simulink model "gm_FP_sub"  (R2023a)
settings: Solver=FixedStepAuto  StartTime=0.0  StopTime=T  RelTol=1e-3  EnableMultiTasking=on
undefined symbols (not defined in the file or in its folder): Ts
libraries: My_FI_Operations x114, simulink x1
(part 2 of 2)

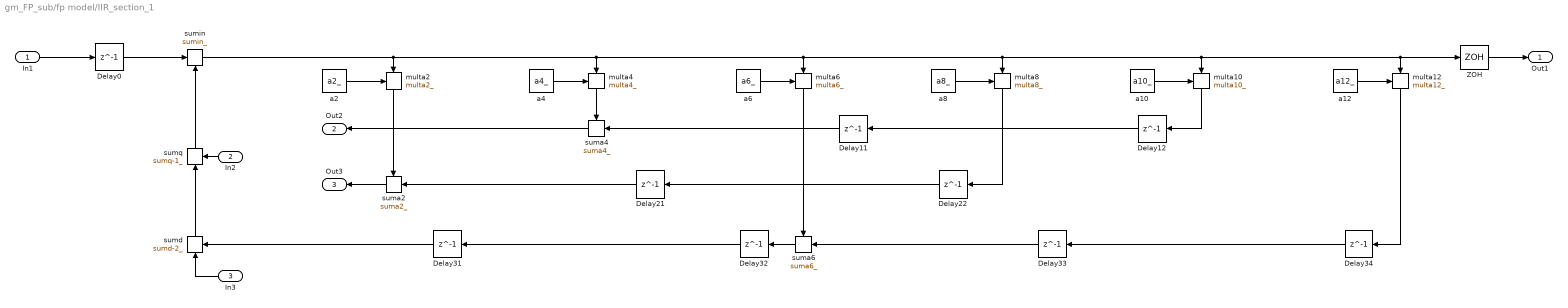
== system gm_FP_sub/fp model/IIR_section_1 ==
  In1 : Inport
  In2 : Inport  Port=2
  In3 : Inport  Port=3
  Delay{0,11..12,21..22,31..34} (9 alike) : Delay  DelayLength=1  SampleTime=3*Ts
  ZOH : ZeroOrderHold  SampleTime=3*Ts
  a10 : My_FI_Operations/a10_  SystemSampleTime=-1  VariantActivationTime=update diagram  Latency=0  AutoFrameSizeCalculation=off
  a12 : My_FI_Operations/a12_  SystemSampleTime=-1  VariantActivationTime=update diagram  Latency=0  AutoFrameSizeCalculation=off
  a2 : My_FI_Operations/a2_  SystemSampleTime=-1  VariantActivationTime=update diagram  Latency=0  AutoFrameSizeCalculation=off
  a4 : My_FI_Operations/a4_  SystemSampleTime=-1  VariantActivationTime=update diagram  Latency=0  AutoFrameSizeCalculation=off
  a6 : My_FI_Operations/a6_  SystemSampleTime=-1  VariantActivationTime=update diagram  Latency=0  AutoFrameSizeCalculation=off
  a8 : My_FI_Operations/a8_  SystemSampleTime=-1  VariantActivationTime=update diagram  Latency=0  AutoFrameSizeCalculation=off
  multa10 : My_FI_Operations/multa10_  SystemSampleTime=-1  VariantActivationTime=update diagram  Latency=0  AutoFrameSizeCalculation=off
      settings: PortSchema="{\"entries\":[{\"content\":{\"sides\":[{\"content\":{\"connectorIds\":[\"In1\"]},\"type\":\"ConnectorPlacement.EquallySpacedRectSide\",\"uuid\":\"423828e0-6700-4575-ac06-a5fb7cb5569f\"},{\"content\":{\"connectorIds\":[],\"side\":\"RIGHT\"},\"type\":\"ConnectorPlacement.EquallySpacedRectSide\",\"uuid\":\"a42db842-eb55-44f2-8f04-0144bc45d908\"},{\"content\":{\"connectorIds\":[\"In2\"],\"side\":\"TOP\"},\"type\":\"ConnectorPlacement.EquallySpacedRectSide\",\"uuid\":\"eef5137d-31f0-46b4-a53b-5aa31464a7f9\"},{\"content\":{\"connectorIds\":[\"Out1\"],\"side\":\"BOTTOM\"},\"type\":\"ConnectorPlacement.EquallySpacedRectSide\",\"uuid\":\"0c804fa9-8d94-49f3-91d8-5fb511150c33\"}]},\"type\":\"ConnectorPlacement.EquallySpacedConnector\",\"uuid\":\"7dd7fe03-b221-4701-a7b2-6552f08320da\"}],\"packageUris\":[\"http://schema.mathworks.com/mf0/Connector/R2020b\"],\"version\":\"1.0\"}"
  multa12 : My_FI_Operations/multa12_  SystemSampleTime=-1  VariantActivationTime=update diagram  Latency=0  AutoFrameSizeCalculation=off
      settings: PortSchema="{\"entries\":[{\"content\":{\"sides\":[{\"content\":{\"connectorIds\":[\"In1\"]},\"type\":\"ConnectorPlacement.EquallySpacedRectSide\",\"uuid\":\"423828e0-6700-4575-ac06-a5fb7cb5569f\"},{\"content\":{\"connectorIds\":[],\"side\":\"RIGHT\"},\"type\":\"ConnectorPlacement.EquallySpacedRectSide\",\"uuid\":\"a42db842-eb55-44f2-8f04-0144bc45d908\"},{\"content\":{\"connectorIds\":[\"In2\"],\"side\":\"TOP\"},\"type\":\"ConnectorPlacement.EquallySpacedRectSide\",\"uuid\":\"eef5137d-31f0-46b4-a53b-5aa31464a7f9\"},{\"content\":{\"connectorIds\":[\"Out1\"],\"side\":\"BOTTOM\"},\"type\":\"ConnectorPlacement.EquallySpacedRectSide\",\"uuid\":\"8449918d-02c6-4967-8b4f-9e277713318d\"}]},\"type\":\"ConnectorPlacement.EquallySpacedConnector\",\"uuid\":\"7dd7fe03-b221-4701-a7b2-6552f08320da\"}],\"packageUris\":[\"http://schema.mathworks.com/mf0/Connector/R2020b\"],\"version\":\"1.0\"}"
  multa2 : My_FI_Operations/multa2_  SystemSampleTime=-1  VariantActivationTime=update diagram  Latency=0  AutoFrameSizeCalculation=off
      settings: PortSchema="{\"entries\":[{\"content\":{\"sides\":[{\"content\":{\"connectorIds\":[\"In1\"]},\"type\":\"ConnectorPlacement.EquallySpacedRectSide\",\"uuid\":\"423828e0-6700-4575-ac06-a5fb7cb5569f\"},{\"content\":{\"connectorIds\":[],\"side\":\"RIGHT\"},\"type\":\"ConnectorPlacement.EquallySpacedRectSide\",\"uuid\":\"a42db842-eb55-44f2-8f04-0144bc45d908\"},{\"content\":{\"connectorIds\":[\"In2\"],\"side\":\"TOP\"},\"type\":\"ConnectorPlacement.EquallySpacedRectSide\",\"uuid\":\"eef5137d-31f0-46b4-a53b-5aa31464a7f9\"},{\"content\":{\"connectorIds\":[\"Out1\"],\"side\":\"BOTTOM\"},\"type\":\"ConnectorPlacement.EquallySpacedRectSide\",\"uuid\":\"55d96b2a-2b7e-4fdf-a401-8e78f7d2a1aa\"}]},\"type\":\"ConnectorPlacement.EquallySpacedConnector\",\"uuid\":\"7dd7fe03-b221-4701-a7b2-6552f08320da\"}],\"packageUris\":[\"http://schema.mathworks.com/mf0/Connector/R2020b\"],\"version\":\"1.0\"}"
  multa4 : My_FI_Operations/multa4_  SystemSampleTime=-1  VariantActivationTime=update diagram  Latency=0  AutoFrameSizeCalculation=off
      settings: PortSchema="{\"entries\":[{\"content\":{\"sides\":[{\"content\":{\"connectorIds\":[\"In1\"]},\"type\":\"ConnectorPlacement.EquallySpacedRectSide\",\"uuid\":\"423828e0-6700-4575-ac06-a5fb7cb5569f\"},{\"content\":{\"connectorIds\":[],\"side\":\"RIGHT\"},\"type\":\"ConnectorPlacement.EquallySpacedRectSide\",\"uuid\":\"a42db842-eb55-44f2-8f04-0144bc45d908\"},{\"content\":{\"connectorIds\":[\"In2\"],\"side\":\"TOP\"},\"type\":\"ConnectorPlacement.EquallySpacedRectSide\",\"uuid\":\"eef5137d-31f0-46b4-a53b-5aa31464a7f9\"},{\"content\":{\"connectorIds\":[\"Out1\"],\"side\":\"BOTTOM\"},\"type\":\"ConnectorPlacement.EquallySpacedRectSide\",\"uuid\":\"24a9476e-4370-431a-bbc5-245c90c7a6e7\"}]},\"type\":\"ConnectorPlacement.EquallySpacedConnector\",\"uuid\":\"7dd7fe03-b221-4701-a7b2-6552f08320da\"}],\"packageUris\":[\"http://schema.mathworks.com/mf0/Connector/R2020b\"],\"version\":\"1.0\"}"
  multa6 : My_FI_Operations/multa6_  SystemSampleTime=-1  VariantActivationTime=update diagram  Latency=0  AutoFrameSizeCalculation=off
      settings: PortSchema="{\"entries\":[{\"content\":{\"sides\":[{\"content\":{\"connectorIds\":[\"In1\"]},\"type\":\"ConnectorPlacement.EquallySpacedRectSide\",\"uuid\":\"423828e0-6700-4575-ac06-a5fb7cb5569f\"},{\"content\":{\"connectorIds\":[],\"side\":\"RIGHT\"},\"type\":\"ConnectorPlacement.EquallySpacedRectSide\",\"uuid\":\"a42db842-eb55-44f2-8f04-0144bc45d908\"},{\"content\":{\"connectorIds\":[\"In2\"],\"side\":\"TOP\"},\"type\":\"ConnectorPlacement.EquallySpacedRectSide\",\"uuid\":\"eef5137d-31f0-46b4-a53b-5aa31464a7f9\"},{\"content\":{\"connectorIds\":[\"Out1\"],\"side\":\"BOTTOM\"},\"type\":\"ConnectorPlacement.EquallySpacedRectSide\",\"uuid\":\"47329aef-84bb-47a0-9b32-b12909a392a1\"}]},\"type\":\"ConnectorPlacement.EquallySpacedConnector\",\"uuid\":\"7dd7fe03-b221-4701-a7b2-6552f08320da\"}],\"packageUris\":[\"http://schema.mathworks.com/mf0/Connector/R2020b\"],\"version\":\"1.0\"}"
  multa8 : My_FI_Operations/multa8_  SystemSampleTime=-1  VariantActivationTime=update diagram  Latency=0  AutoFrameSizeCalculation=off
      settings: PortSchema="{\"entries\":[{\"content\":{\"sides\":[{\"content\":{\"connectorIds\":[\"In1\"]},\"type\":\"ConnectorPlacement.EquallySpacedRectSide\",\"uuid\":\"423828e0-6700-4575-ac06-a5fb7cb5569f\"},{\"content\":{\"connectorIds\":[],\"side\":\"RIGHT\"},\"type\":\"ConnectorPlacement.EquallySpacedRectSide\",\"uuid\":\"a42db842-eb55-44f2-8f04-0144bc45d908\"},{\"content\":{\"connectorIds\":[\"In2\"],\"side\":\"TOP\"},\"type\":\"ConnectorPlacement.EquallySpacedRectSide\",\"uuid\":\"eef5137d-31f0-46b4-a53b-5aa31464a7f9\"},{\"content\":{\"connectorIds\":[\"Out1\"],\"side\":\"BOTTOM\"},\"type\":\"ConnectorPlacement.EquallySpacedRectSide\",\"uuid\":\"5c073f60-f22f-4cd7-abc5-d0d5f88f0213\"}]},\"type\":\"ConnectorPlacement.EquallySpacedConnector\",\"uuid\":\"7dd7fe03-b221-4701-a7b2-6552f08320da\"}],\"packageUris\":[\"http://schema.mathworks.com/mf0/Connector/R2020b\"],\"version\":\"1.0\"}"
  suma2 : My_FI_Operations/suma2_  SystemSampleTime=-1  VariantActivationTime=update diagram  Latency=0  AutoFrameSizeCalculation=off
      settings: PortSchema="{\"entries\":[{\"content\":{\"sides\":[{\"content\":{\"connectorIds\":[\"Out1\"]},\"type\":\"ConnectorPlacement.EquallySpacedRectSide\",\"uuid\":\"423828e0-6700-4575-ac06-a5fb7cb5569f\"},{\"content\":{\"connectorIds\":[\"In2\"],\"side\":\"RIGHT\"},\"type\":\"ConnectorPlacement.EquallySpacedRectSide\",\"uuid\":\"a42db842-eb55-44f2-8f04-0144bc45d908\"},{\"content\":{\"connectorIds\":[\"In1\"],\"side\":\"TOP\"},\"type\":\"ConnectorPlacement.EquallySpacedRectSide\",\"uuid\":\"eef5137d-31f0-46b4-a53b-5aa31464a7f9\"}]},\"type\":\"ConnectorPlacement.EquallySpacedConnector\",\"uuid\":\"7dd7fe03-b221-4701-a7b2-6552f08320da\"}],\"packageUris\":[\"http://schema.mathworks.com/mf0/Connector/R2020b\"],\"version\":\"1.0\"}"
  suma4 : My_FI_Operations/suma4_  SystemSampleTime=-1  VariantActivationTime=update diagram  Latency=0  AutoFrameSizeCalculation=off
      settings: PortSchema="{\"entries\":[{\"content\":{\"sides\":[{\"content\":{\"connectorIds\":[\"Out1\"]},\"type\":\"ConnectorPlacement.EquallySpacedRectSide\",\"uuid\":\"423828e0-6700-4575-ac06-a5fb7cb5569f\"},{\"content\":{\"connectorIds\":[\"In2\"],\"side\":\"RIGHT\"},\"type\":\"ConnectorPlacement.EquallySpacedRectSide\",\"uuid\":\"a42db842-eb55-44f2-8f04-0144bc45d908\"},{\"content\":{\"connectorIds\":[\"In1\"],\"side\":\"TOP\"},\"type\":\"ConnectorPlacement.EquallySpacedRectSide\",\"uuid\":\"eef5137d-31f0-46b4-a53b-5aa31464a7f9\"}]},\"type\":\"ConnectorPlacement.EquallySpacedConnector\",\"uuid\":\"7dd7fe03-b221-4701-a7b2-6552f08320da\"}],\"packageUris\":[\"http://schema.mathworks.com/mf0/Connector/R2020b\"],\"version\":\"1.0\"}"
  suma6 : My_FI_Operations/suma6_  SystemSampleTime=-1  VariantActivationTime=update diagram  Latency=0  AutoFrameSizeCalculation=off
      settings: PortSchema="{\"entries\":[{\"content\":{\"sides\":[{\"content\":{\"connectorIds\":[\"Out1\"]},\"type\":\"ConnectorPlacement.EquallySpacedRectSide\",\"uuid\":\"423828e0-6700-4575-ac06-a5fb7cb5569f\"},{\"content\":{\"connectorIds\":[\"In2\"],\"side\":\"RIGHT\"},\"type\":\"ConnectorPlacement.EquallySpacedRectSide\",\"uuid\":\"a42db842-eb55-44f2-8f04-0144bc45d908\"},{\"content\":{\"connectorIds\":[\"In1\"],\"side\":\"TOP\"},\"type\":\"ConnectorPlacement.EquallySpacedRectSide\",\"uuid\":\"eef5137d-31f0-46b4-a53b-5aa31464a7f9\"}]},\"type\":\"ConnectorPlacement.EquallySpacedConnector\",\"uuid\":\"7dd7fe03-b221-4701-a7b2-6552f08320da\"}],\"packageUris\":[\"http://schema.mathworks.com/mf0/Connector/R2020b\"],\"version\":\"1.0\"}"
  sumd : My_FI_Operations/sumd-2_  SystemSampleTime=-1  VariantActivationTime=update diagram  Latency=0  AutoFrameSizeCalculation=off
      settings: PortSchema="{\"entries\":[{\"content\":{\"sides\":[{\"content\":{\"connectorIds\":[]},\"type\":\"ConnectorPlacement.EquallySpacedRectSide\",\"uuid\":\"423828e0-6700-4575-ac06-a5fb7cb5569f\"},{\"content\":{\"connectorIds\":[\"In2\"],\"side\":\"RIGHT\"},\"type\":\"ConnectorPlacement.EquallySpacedRectSide\",\"uuid\":\"a42db842-eb55-44f2-8f04-0144bc45d908\"},{\"content\":{\"connectorIds\":[\"Out1\"],\"side\":\"TOP\"},\"type\":\"ConnectorPlacement.EquallySpacedRectSide\",\"uuid\":\"eef5137d-31f0-46b4-a53b-5aa31464a7f9\"},{\"content\":{\"connectorIds\":[\"In1\"],\"side\":\"BOTTOM\"},\"type\":\"ConnectorPlacement.EquallySpacedRectSide\",\"uuid\":\"0a29e77a-4bdf-45d0-8a25-1103c3446174\"}]},\"type\":\"ConnectorPlacement.EquallySpacedConnector\",\"uuid\":\"7dd7fe03-b221-4701-a7b2-6552f08320da\"}],\"packageUris\":[\"http://schema.mathworks.com/mf0/Connector/R2020b\"],\"version\":\"1.0\"}"
  sumin : My_FI_Operations/sumin_  SystemSampleTime=-1  VariantActivationTime=update diagram  Latency=0  AutoFrameSizeCalculation=off
      settings: PortSchema="{\"entries\":[{\"content\":{\"sides\":[{\"content\":{\"connectorIds\":[\"In1\"]},\"type\":\"ConnectorPlacement.EquallySpacedRectSide\",\"uuid\":\"423828e0-6700-4575-ac06-a5fb7cb5569f\"},{\"content\":{\"connectorIds\":[\"Out1\"],\"side\":\"RIGHT\"},\"type\":\"ConnectorPlacement.EquallySpacedRectSide\",\"uuid\":\"a42db842-eb55-44f2-8f04-0144bc45d908\"},{\"content\":{\"connectorIds\":[],\"side\":\"TOP\"},\"type\":\"ConnectorPlacement.EquallySpacedRectSide\",\"uuid\":\"eef5137d-31f0-46b4-a53b-5aa31464a7f9\"},{\"content\":{\"connectorIds\":[\"In2\"],\"side\":\"BOTTOM\"},\"type\":\"ConnectorPlacement.EquallySpacedRectSide\",\"uuid\":\"f3760898-0e2b-4385-8757-2cc61988fa54\"}]},\"type\":\"ConnectorPlacement.EquallySpacedConnector\",\"uuid\":\"7dd7fe03-b221-4701-a7b2-6552f08320da\"}],\"packageUris\":[\"http://schema.mathworks.com/mf0/Connector/R2020b\"],\"version\":\"1.0\"}"
  sumq : My_FI_Operations/sumq-1_  SystemSampleTime=-1  VariantActivationTime=update diagram  Latency=0  AutoFrameSizeCalculation=off
      settings: PortSchema="{\"entries\":[{\"content\":{\"sides\":[{\"content\":{\"connectorIds\":[]},\"type\":\"ConnectorPlacement.EquallySpacedRectSide\",\"uuid\":\"423828e0-6700-4575-ac06-a5fb7cb5569f\"},{\"content\":{\"connectorIds\":[\"In2\"],\"side\":\"RIGHT\"},\"type\":\"ConnectorPlacement.EquallySpacedRectSide\",\"uuid\":\"a42db842-eb55-44f2-8f04-0144bc45d908\"},{\"content\":{\"connectorIds\":[\"Out1\"],\"side\":\"TOP\"},\"type\":\"ConnectorPlacement.EquallySpacedRectSide\",\"uuid\":\"eef5137d-31f0-46b4-a53b-5aa31464a7f9\"},{\"content\":{\"connectorIds\":[\"In1\"],\"side\":\"BOTTOM\"},\"type\":\"ConnectorPlacement.EquallySpacedRectSide\",\"uuid\":\"2873f229-5340-47da-9b40-109923f96826\"}]},\"type\":\"ConnectorPlacement.EquallySpacedConnector\",\"uuid\":\"7dd7fe03-b221-4701-a7b2-6552f08320da\"}],\"packageUris\":[\"http://schema.mathworks.com/mf0/Connector/R2020b\"],\"version\":\"1.0\"}"
  Out1 : Outport
  Out2 : Outport  Port=2
  Out3 : Outport  Port=3
  wires:
  suma4/1 -> Out2/1
  suma2/1 -> Out3/1
  In3/1 -> sumd/1
  In1/1 -> Delay0/1
  In2/1 -> sumq/2
  a6/1 -> multa6/1
  sumq/1 -> sumin/2
  multa8/1 -> Delay22/1
  multa10/1 -> Delay12/1
  Delay11/1 -> suma4/2
  suma6/1 -> Delay32/1
  a8/1 -> multa8/1
  Delay34/1 -> Delay33/1
  multa2/1 -> suma2/1
  multa12/1 -> Delay34/1
  a4/1 -> multa4/1
  a10/1 -> multa10/1
  multa6/1 -> suma6/1
  ZOH/1 -> Out1/1
  Delay12/1 -> Delay11/1
  multa4/1 -> suma4/1
  a2/1 -> multa2/1
  sumd/1 -> sumq/1
  Delay21/1 -> suma2/2
  Delay32/1 -> Delay31/1
  Delay33/1 -> suma6/2
  sumin/1 -> ZOH/1, multa12/2, multa10/2, multa8/2, multa6/2, multa4/2, multa2/2
  Delay31/1 -> sumd/2
  Delay22/1 -> Delay21/1
  a12/1 -> multa12/1
  Delay0/1 -> sumin/1

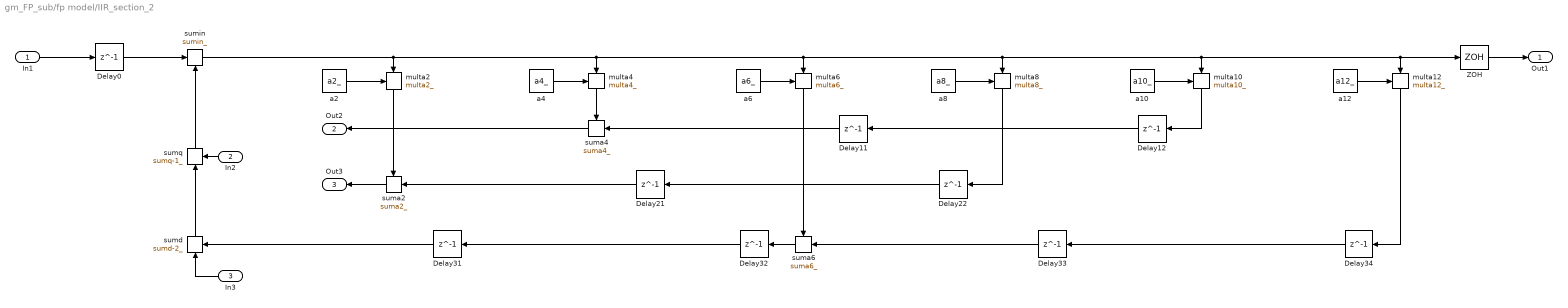
== system gm_FP_sub/fp model/IIR_section_2 ==
  In1 : Inport
  In2 : Inport  Port=2
  In3 : Inport  Port=3
  Delay{0,11..12,21..22,31..34} (9 alike) : Delay  DelayLength=1  SampleTime=3*Ts
  ZOH : ZeroOrderHold  SampleTime=3*Ts
  a10 : My_FI_Operations/a10_  SystemSampleTime=-1  VariantActivationTime=update diagram  Latency=0  AutoFrameSizeCalculation=off
  a12 : My_FI_Operations/a12_  SystemSampleTime=-1  VariantActivationTime=update diagram  Latency=0  AutoFrameSizeCalculation=off
  a2 : My_FI_Operations/a2_  SystemSampleTime=-1  VariantActivationTime=update diagram  Latency=0  AutoFrameSizeCalculation=off
  a4 : My_FI_Operations/a4_  SystemSampleTime=-1  VariantActivationTime=update diagram  Latency=0  AutoFrameSizeCalculation=off
  a6 : My_FI_Operations/a6_  SystemSampleTime=-1  VariantActivationTime=update diagram  Latency=0  AutoFrameSizeCalculation=off
  a8 : My_FI_Operations/a8_  SystemSampleTime=-1  VariantActivationTime=update diagram  Latency=0  AutoFrameSizeCalculation=off
  multa10 : My_FI_Operations/multa10_  SystemSampleTime=-1  VariantActivationTime=update diagram  Latency=0  AutoFrameSizeCalculation=off
      settings: PortSchema="{\"entries\":[{\"content\":{\"sides\":[{\"content\":{\"connectorIds\":[\"In1\"]},\"type\":\"ConnectorPlacement.EquallySpacedRectSide\",\"uuid\":\"423828e0-6700-4575-ac06-a5fb7cb5569f\"},{\"content\":{\"connectorIds\":[],\"side\":\"RIGHT\"},\"type\":\"ConnectorPlacement.EquallySpacedRectSide\",\"uuid\":\"a42db842-eb55-44f2-8f04-0144bc45d908\"},{\"content\":{\"connectorIds\":[\"In2\"],\"side\":\"TOP\"},\"type\":\"ConnectorPlacement.EquallySpacedRectSide\",\"uuid\":\"eef5137d-31f0-46b4-a53b-5aa31464a7f9\"},{\"content\":{\"connectorIds\":[\"Out1\"],\"side\":\"BOTTOM\"},\"type\":\"ConnectorPlacement.EquallySpacedRectSide\",\"uuid\":\"0c804fa9-8d94-49f3-91d8-5fb511150c33\"}]},\"type\":\"ConnectorPlacement.EquallySpacedConnector\",\"uuid\":\"7dd7fe03-b221-4701-a7b2-6552f08320da\"}],\"packageUris\":[\"http://schema.mathworks.com/mf0/Connector/R2020b\"],\"version\":\"1.0\"}"
  multa12 : My_FI_Operations/multa12_  SystemSampleTime=-1  VariantActivationTime=update diagram  Latency=0  AutoFrameSizeCalculation=off
      settings: PortSchema="{\"entries\":[{\"content\":{\"sides\":[{\"content\":{\"connectorIds\":[\"In1\"]},\"type\":\"ConnectorPlacement.EquallySpacedRectSide\",\"uuid\":\"423828e0-6700-4575-ac06-a5fb7cb5569f\"},{\"content\":{\"connectorIds\":[],\"side\":\"RIGHT\"},\"type\":\"ConnectorPlacement.EquallySpacedRectSide\",\"uuid\":\"a42db842-eb55-44f2-8f04-0144bc45d908\"},{\"content\":{\"connectorIds\":[\"In2\"],\"side\":\"TOP\"},\"type\":\"ConnectorPlacement.EquallySpacedRectSide\",\"uuid\":\"eef5137d-31f0-46b4-a53b-5aa31464a7f9\"},{\"content\":{\"connectorIds\":[\"Out1\"],\"side\":\"BOTTOM\"},\"type\":\"ConnectorPlacement.EquallySpacedRectSide\",\"uuid\":\"8449918d-02c6-4967-8b4f-9e277713318d\"}]},\"type\":\"ConnectorPlacement.EquallySpacedConnector\",\"uuid\":\"7dd7fe03-b221-4701-a7b2-6552f08320da\"}],\"packageUris\":[\"http://schema.mathworks.com/mf0/Connector/R2020b\"],\"version\":\"1.0\"}"
  multa2 : My_FI_Operations/multa2_  SystemSampleTime=-1  VariantActivationTime=update diagram  Latency=0  AutoFrameSizeCalculation=off
      settings: PortSchema="{\"entries\":[{\"content\":{\"sides\":[{\"content\":{\"connectorIds\":[\"In1\"]},\"type\":\"ConnectorPlacement.EquallySpacedRectSide\",\"uuid\":\"423828e0-6700-4575-ac06-a5fb7cb5569f\"},{\"content\":{\"connectorIds\":[],\"side\":\"RIGHT\"},\"type\":\"ConnectorPlacement.EquallySpacedRectSide\",\"uuid\":\"a42db842-eb55-44f2-8f04-0144bc45d908\"},{\"content\":{\"connectorIds\":[\"In2\"],\"side\":\"TOP\"},\"type\":\"ConnectorPlacement.EquallySpacedRectSide\",\"uuid\":\"eef5137d-31f0-46b4-a53b-5aa31464a7f9\"},{\"content\":{\"connectorIds\":[\"Out1\"],\"side\":\"BOTTOM\"},\"type\":\"ConnectorPlacement.EquallySpacedRectSide\",\"uuid\":\"55d96b2a-2b7e-4fdf-a401-8e78f7d2a1aa\"}]},\"type\":\"ConnectorPlacement.EquallySpacedConnector\",\"uuid\":\"7dd7fe03-b221-4701-a7b2-6552f08320da\"}],\"packageUris\":[\"http://schema.mathworks.com/mf0/Connector/R2020b\"],\"version\":\"1.0\"}"
  multa4 : My_FI_Operations/multa4_  SystemSampleTime=-1  VariantActivationTime=update diagram  Latency=0  AutoFrameSizeCalculation=off
      settings: PortSchema="{\"entries\":[{\"content\":{\"sides\":[{\"content\":{\"connectorIds\":[\"In1\"]},\"type\":\"ConnectorPlacement.EquallySpacedRectSide\",\"uuid\":\"423828e0-6700-4575-ac06-a5fb7cb5569f\"},{\"content\":{\"connectorIds\":[],\"side\":\"RIGHT\"},\"type\":\"ConnectorPlacement.EquallySpacedRectSide\",\"uuid\":\"a42db842-eb55-44f2-8f04-0144bc45d908\"},{\"content\":{\"connectorIds\":[\"In2\"],\"side\":\"TOP\"},\"type\":\"ConnectorPlacement.EquallySpacedRectSide\",\"uuid\":\"eef5137d-31f0-46b4-a53b-5aa31464a7f9\"},{\"content\":{\"connectorIds\":[\"Out1\"],\"side\":\"BOTTOM\"},\"type\":\"ConnectorPlacement.EquallySpacedRectSide\",\"uuid\":\"24a9476e-4370-431a-bbc5-245c90c7a6e7\"}]},\"type\":\"ConnectorPlacement.EquallySpacedConnector\",\"uuid\":\"7dd7fe03-b221-4701-a7b2-6552f08320da\"}],\"packageUris\":[\"http://schema.mathworks.com/mf0/Connector/R2020b\"],\"version\":\"1.0\"}"
  multa6 : My_FI_Operations/multa6_  SystemSampleTime=-1  VariantActivationTime=update diagram  Latency=0  AutoFrameSizeCalculation=off
      settings: PortSchema="{\"entries\":[{\"content\":{\"sides\":[{\"content\":{\"connectorIds\":[\"In1\"]},\"type\":\"ConnectorPlacement.EquallySpacedRectSide\",\"uuid\":\"423828e0-6700-4575-ac06-a5fb7cb5569f\"},{\"content\":{\"connectorIds\":[],\"side\":\"RIGHT\"},\"type\":\"ConnectorPlacement.EquallySpacedRectSide\",\"uuid\":\"a42db842-eb55-44f2-8f04-0144bc45d908\"},{\"content\":{\"connectorIds\":[\"In2\"],\"side\":\"TOP\"},\"type\":\"ConnectorPlacement.EquallySpacedRectSide\",\"uuid\":\"eef5137d-31f0-46b4-a53b-5aa31464a7f9\"},{\"content\":{\"connectorIds\":[\"Out1\"],\"side\":\"BOTTOM\"},\"type\":\"ConnectorPlacement.EquallySpacedRectSide\",\"uuid\":\"47329aef-84bb-47a0-9b32-b12909a392a1\"}]},\"type\":\"ConnectorPlacement.EquallySpacedConnector\",\"uuid\":\"7dd7fe03-b221-4701-a7b2-6552f08320da\"}],\"packageUris\":[\"http://schema.mathworks.com/mf0/Connector/R2020b\"],\"version\":\"1.0\"}"
  multa8 : My_FI_Operations/multa8_  SystemSampleTime=-1  VariantActivationTime=update diagram  Latency=0  AutoFrameSizeCalculation=off
      settings: PortSchema="{\"entries\":[{\"content\":{\"sides\":[{\"content\":{\"connectorIds\":[\"In1\"]},\"type\":\"ConnectorPlacement.EquallySpacedRectSide\",\"uuid\":\"423828e0-6700-4575-ac06-a5fb7cb5569f\"},{\"content\":{\"connectorIds\":[],\"side\":\"RIGHT\"},\"type\":\"ConnectorPlacement.EquallySpacedRectSide\",\"uuid\":\"a42db842-eb55-44f2-8f04-0144bc45d908\"},{\"content\":{\"connectorIds\":[\"In2\"],\"side\":\"TOP\"},\"type\":\"ConnectorPlacement.EquallySpacedRectSide\",\"uuid\":\"eef5137d-31f0-46b4-a53b-5aa31464a7f9\"},{\"content\":{\"connectorIds\":[\"Out1\"],\"side\":\"BOTTOM\"},\"type\":\"ConnectorPlacement.EquallySpacedRectSide\",\"uuid\":\"5c073f60-f22f-4cd7-abc5-d0d5f88f0213\"}]},\"type\":\"ConnectorPlacement.EquallySpacedConnector\",\"uuid\":\"7dd7fe03-b221-4701-a7b2-6552f08320da\"}],\"packageUris\":[\"http://schema.mathworks.com/mf0/Connector/R2020b\"],\"version\":\"1.0\"}"
  suma2 : My_FI_Operations/suma2_  SystemSampleTime=-1  VariantActivationTime=update diagram  Latency=0  AutoFrameSizeCalculation=off
      settings: PortSchema="{\"entries\":[{\"content\":{\"sides\":[{\"content\":{\"connectorIds\":[\"Out1\"]},\"type\":\"ConnectorPlacement.EquallySpacedRectSide\",\"uuid\":\"423828e0-6700-4575-ac06-a5fb7cb5569f\"},{\"content\":{\"connectorIds\":[\"In2\"],\"side\":\"RIGHT\"},\"type\":\"ConnectorPlacement.EquallySpacedRectSide\",\"uuid\":\"a42db842-eb55-44f2-8f04-0144bc45d908\"},{\"content\":{\"connectorIds\":[\"In1\"],\"side\":\"TOP\"},\"type\":\"ConnectorPlacement.EquallySpacedRectSide\",\"uuid\":\"eef5137d-31f0-46b4-a53b-5aa31464a7f9\"}]},\"type\":\"ConnectorPlacement.EquallySpacedConnector\",\"uuid\":\"7dd7fe03-b221-4701-a7b2-6552f08320da\"}],\"packageUris\":[\"http://schema.mathworks.com/mf0/Connector/R2020b\"],\"version\":\"1.0\"}"
  suma4 : My_FI_Operations/suma4_  SystemSampleTime=-1  VariantActivationTime=update diagram  Latency=0  AutoFrameSizeCalculation=off
      settings: PortSchema="{\"entries\":[{\"content\":{\"sides\":[{\"content\":{\"connectorIds\":[\"Out1\"]},\"type\":\"ConnectorPlacement.EquallySpacedRectSide\",\"uuid\":\"423828e0-6700-4575-ac06-a5fb7cb5569f\"},{\"content\":{\"connectorIds\":[\"In2\"],\"side\":\"RIGHT\"},\"type\":\"ConnectorPlacement.EquallySpacedRectSide\",\"uuid\":\"a42db842-eb55-44f2-8f04-0144bc45d908\"},{\"content\":{\"connectorIds\":[\"In1\"],\"side\":\"TOP\"},\"type\":\"ConnectorPlacement.EquallySpacedRectSide\",\"uuid\":\"eef5137d-31f0-46b4-a53b-5aa31464a7f9\"}]},\"type\":\"ConnectorPlacement.EquallySpacedConnector\",\"uuid\":\"7dd7fe03-b221-4701-a7b2-6552f08320da\"}],\"packageUris\":[\"http://schema.mathworks.com/mf0/Connector/R2020b\"],\"version\":\"1.0\"}"
  suma6 : My_FI_Operations/suma6_  SystemSampleTime=-1  VariantActivationTime=update diagram  Latency=0  AutoFrameSizeCalculation=off
      settings: PortSchema="{\"entries\":[{\"content\":{\"sides\":[{\"content\":{\"connectorIds\":[\"Out1\"]},\"type\":\"ConnectorPlacement.EquallySpacedRectSide\",\"uuid\":\"423828e0-6700-4575-ac06-a5fb7cb5569f\"},{\"content\":{\"connectorIds\":[\"In2\"],\"side\":\"RIGHT\"},\"type\":\"ConnectorPlacement.EquallySpacedRectSide\",\"uuid\":\"a42db842-eb55-44f2-8f04-0144bc45d908\"},{\"content\":{\"connectorIds\":[\"In1\"],\"side\":\"TOP\"},\"type\":\"ConnectorPlacement.EquallySpacedRectSide\",\"uuid\":\"eef5137d-31f0-46b4-a53b-5aa31464a7f9\"}]},\"type\":\"ConnectorPlacement.EquallySpacedConnector\",\"uuid\":\"7dd7fe03-b221-4701-a7b2-6552f08320da\"}],\"packageUris\":[\"http://schema.mathworks.com/mf0/Connector/R2020b\"],\"version\":\"1.0\"}"
  sumd : My_FI_Operations/sumd-2_  SystemSampleTime=-1  VariantActivationTime=update diagram  Latency=0  AutoFrameSizeCalculation=off
      settings: PortSchema="{\"entries\":[{\"content\":{\"sides\":[{\"content\":{\"connectorIds\":[]},\"type\":\"ConnectorPlacement.EquallySpacedRectSide\",\"uuid\":\"423828e0-6700-4575-ac06-a5fb7cb5569f\"},{\"content\":{\"connectorIds\":[\"In2\"],\"side\":\"RIGHT\"},\"type\":\"ConnectorPlacement.EquallySpacedRectSide\",\"uuid\":\"a42db842-eb55-44f2-8f04-0144bc45d908\"},{\"content\":{\"connectorIds\":[\"Out1\"],\"side\":\"TOP\"},\"type\":\"ConnectorPlacement.EquallySpacedRectSide\",\"uuid\":\"eef5137d-31f0-46b4-a53b-5aa31464a7f9\"},{\"content\":{\"connectorIds\":[\"In1\"],\"side\":\"BOTTOM\"},\"type\":\"ConnectorPlacement.EquallySpacedRectSide\",\"uuid\":\"0a29e77a-4bdf-45d0-8a25-1103c3446174\"}]},\"type\":\"ConnectorPlacement.EquallySpacedConnector\",\"uuid\":\"7dd7fe03-b221-4701-a7b2-6552f08320da\"}],\"packageUris\":[\"http://schema.mathworks.com/mf0/Connector/R2020b\"],\"version\":\"1.0\"}"
  sumin : My_FI_Operations/sumin_  SystemSampleTime=-1  VariantActivationTime=update diagram  Latency=0  AutoFrameSizeCalculation=off
      settings: PortSchema="{\"entries\":[{\"content\":{\"sides\":[{\"content\":{\"connectorIds\":[\"In1\"]},\"type\":\"ConnectorPlacement.EquallySpacedRectSide\",\"uuid\":\"423828e0-6700-4575-ac06-a5fb7cb5569f\"},{\"content\":{\"connectorIds\":[\"Out1\"],\"side\":\"RIGHT\"},\"type\":\"ConnectorPlacement.EquallySpacedRectSide\",\"uuid\":\"a42db842-eb55-44f2-8f04-0144bc45d908\"},{\"content\":{\"connectorIds\":[],\"side\":\"TOP\"},\"type\":\"ConnectorPlacement.EquallySpacedRectSide\",\"uuid\":\"eef5137d-31f0-46b4-a53b-5aa31464a7f9\"},{\"content\":{\"connectorIds\":[\"In2\"],\"side\":\"BOTTOM\"},\"type\":\"ConnectorPlacement.EquallySpacedRectSide\",\"uuid\":\"f3760898-0e2b-4385-8757-2cc61988fa54\"}]},\"type\":\"ConnectorPlacement.EquallySpacedConnector\",\"uuid\":\"7dd7fe03-b221-4701-a7b2-6552f08320da\"}],\"packageUris\":[\"http://schema.mathworks.com/mf0/Connector/R2020b\"],\"version\":\"1.0\"}"
  sumq : My_FI_Operations/sumq-1_  SystemSampleTime=-1  VariantActivationTime=update diagram  Latency=0  AutoFrameSizeCalculation=off
      settings: PortSchema="{\"entries\":[{\"content\":{\"sides\":[{\"content\":{\"connectorIds\":[]},\"type\":\"ConnectorPlacement.EquallySpacedRectSide\",\"uuid\":\"423828e0-6700-4575-ac06-a5fb7cb5569f\"},{\"content\":{\"connectorIds\":[\"In2\"],\"side\":\"RIGHT\"},\"type\":\"ConnectorPlacement.EquallySpacedRectSide\",\"uuid\":\"a42db842-eb55-44f2-8f04-0144bc45d908\"},{\"content\":{\"connectorIds\":[\"Out1\"],\"side\":\"TOP\"},\"type\":\"ConnectorPlacement.EquallySpacedRectSide\",\"uuid\":\"eef5137d-31f0-46b4-a53b-5aa31464a7f9\"},{\"content\":{\"connectorIds\":[\"In1\"],\"side\":\"BOTTOM\"},\"type\":\"ConnectorPlacement.EquallySpacedRectSide\",\"uuid\":\"2873f229-5340-47da-9b40-109923f96826\"}]},\"type\":\"ConnectorPlacement.EquallySpacedConnector\",\"uuid\":\"7dd7fe03-b221-4701-a7b2-6552f08320da\"}],\"packageUris\":[\"http://schema.mathworks.com/mf0/Connector/R2020b\"],\"version\":\"1.0\"}"
  Out1 : Outport
  Out2 : Outport  Port=2
  Out3 : Outport  Port=3
  wires:
  suma4/1 -> Out2/1
  suma2/1 -> Out3/1
  In3/1 -> sumd/1
  In1/1 -> Delay0/1
  In2/1 -> sumq/2
  a6/1 -> multa6/1
  sumq/1 -> sumin/2
  multa8/1 -> Delay22/1
  multa10/1 -> Delay12/1
  Delay11/1 -> suma4/2
  suma6/1 -> Delay32/1
  a8/1 -> multa8/1
  Delay34/1 -> Delay33/1
  multa2/1 -> suma2/1
  multa12/1 -> Delay34/1
  a4/1 -> multa4/1
  a10/1 -> multa10/1
  multa6/1 -> suma6/1
  ZOH/1 -> Out1/1
  Delay12/1 -> Delay11/1
  multa4/1 -> suma4/1
  a2/1 -> multa2/1
  sumd/1 -> sumq/1
  Delay21/1 -> suma2/2
  Delay32/1 -> Delay31/1
  Delay33/1 -> suma6/2
  sumin/1 -> ZOH/1, multa12/2, multa10/2, multa8/2, multa6/2, multa4/2, multa2/2
  Delay31/1 -> sumd/2
  Delay22/1 -> Delay21/1
  a12/1 -> multa12/1
  Delay0/1 -> sumin/1

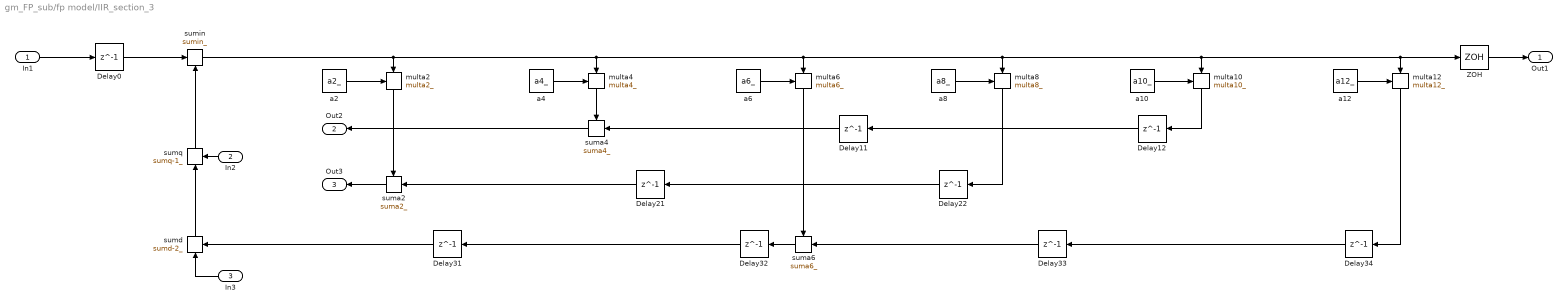
== system gm_FP_sub/fp model/IIR_section_3 ==
  In1 : Inport
  In2 : Inport  Port=2
  In3 : Inport  Port=3
  Delay{0,11..12,21..22,31..34} (9 alike) : Delay  DelayLength=1  SampleTime=3*Ts
  ZOH : ZeroOrderHold  SampleTime=3*Ts
  a10 : My_FI_Operations/a10_  SystemSampleTime=-1  VariantActivationTime=update diagram  Latency=0  AutoFrameSizeCalculation=off
  a12 : My_FI_Operations/a12_  SystemSampleTime=-1  VariantActivationTime=update diagram  Latency=0  AutoFrameSizeCalculation=off
  a2 : My_FI_Operations/a2_  SystemSampleTime=-1  VariantActivationTime=update diagram  Latency=0  AutoFrameSizeCalculation=off
  a4 : My_FI_Operations/a4_  SystemSampleTime=-1  VariantActivationTime=update diagram  Latency=0  AutoFrameSizeCalculation=off
  a6 : My_FI_Operations/a6_  SystemSampleTime=-1  VariantActivationTime=update diagram  Latency=0  AutoFrameSizeCalculation=off
  a8 : My_FI_Operations/a8_  SystemSampleTime=-1  VariantActivationTime=update diagram  Latency=0  AutoFrameSizeCalculation=off
  multa10 : My_FI_Operations/multa10_  SystemSampleTime=-1  VariantActivationTime=update diagram  Latency=0  AutoFrameSizeCalculation=off
      settings: PortSchema="{\"entries\":[{\"content\":{\"sides\":[{\"content\":{\"connectorIds\":[\"In1\"]},\"type\":\"ConnectorPlacement.EquallySpacedRectSide\",\"uuid\":\"423828e0-6700-4575-ac06-a5fb7cb5569f\"},{\"content\":{\"connectorIds\":[],\"side\":\"RIGHT\"},\"type\":\"ConnectorPlacement.EquallySpacedRectSide\",\"uuid\":\"a42db842-eb55-44f2-8f04-0144bc45d908\"},{\"content\":{\"connectorIds\":[\"In2\"],\"side\":\"TOP\"},\"type\":\"ConnectorPlacement.EquallySpacedRectSide\",\"uuid\":\"eef5137d-31f0-46b4-a53b-5aa31464a7f9\"},{\"content\":{\"connectorIds\":[\"Out1\"],\"side\":\"BOTTOM\"},\"type\":\"ConnectorPlacement.EquallySpacedRectSide\",\"uuid\":\"0c804fa9-8d94-49f3-91d8-5fb511150c33\"}]},\"type\":\"ConnectorPlacement.EquallySpacedConnector\",\"uuid\":\"7dd7fe03-b221-4701-a7b2-6552f08320da\"}],\"packageUris\":[\"http://schema.mathworks.com/mf0/Connector/R2020b\"],\"version\":\"1.0\"}"
  multa12 : My_FI_Operations/multa12_  SystemSampleTime=-1  VariantActivationTime=update diagram  Latency=0  AutoFrameSizeCalculation=off
      settings: PortSchema="{\"entries\":[{\"content\":{\"sides\":[{\"content\":{\"connectorIds\":[\"In1\"]},\"type\":\"ConnectorPlacement.EquallySpacedRectSide\",\"uuid\":\"423828e0-6700-4575-ac06-a5fb7cb5569f\"},{\"content\":{\"connectorIds\":[],\"side\":\"RIGHT\"},\"type\":\"ConnectorPlacement.EquallySpacedRectSide\",\"uuid\":\"a42db842-eb55-44f2-8f04-0144bc45d908\"},{\"content\":{\"connectorIds\":[\"In2\"],\"side\":\"TOP\"},\"type\":\"ConnectorPlacement.EquallySpacedRectSide\",\"uuid\":\"eef5137d-31f0-46b4-a53b-5aa31464a7f9\"},{\"content\":{\"connectorIds\":[\"Out1\"],\"side\":\"BOTTOM\"},\"type\":\"ConnectorPlacement.EquallySpacedRectSide\",\"uuid\":\"8449918d-02c6-4967-8b4f-9e277713318d\"}]},\"type\":\"ConnectorPlacement.EquallySpacedConnector\",\"uuid\":\"7dd7fe03-b221-4701-a7b2-6552f08320da\"}],\"packageUris\":[\"http://schema.mathworks.com/mf0/Connector/R2020b\"],\"version\":\"1.0\"}"
  multa2 : My_FI_Operations/multa2_  SystemSampleTime=-1  VariantActivationTime=update diagram  Latency=0  AutoFrameSizeCalculation=off
      settings: PortSchema="{\"entries\":[{\"content\":{\"sides\":[{\"content\":{\"connectorIds\":[\"In1\"]},\"type\":\"ConnectorPlacement.EquallySpacedRectSide\",\"uuid\":\"423828e0-6700-4575-ac06-a5fb7cb5569f\"},{\"content\":{\"connectorIds\":[],\"side\":\"RIGHT\"},\"type\":\"ConnectorPlacement.EquallySpacedRectSide\",\"uuid\":\"a42db842-eb55-44f2-8f04-0144bc45d908\"},{\"content\":{\"connectorIds\":[\"In2\"],\"side\":\"TOP\"},\"type\":\"ConnectorPlacement.EquallySpacedRectSide\",\"uuid\":\"eef5137d-31f0-46b4-a53b-5aa31464a7f9\"},{\"content\":{\"connectorIds\":[\"Out1\"],\"side\":\"BOTTOM\"},\"type\":\"ConnectorPlacement.EquallySpacedRectSide\",\"uuid\":\"55d96b2a-2b7e-4fdf-a401-8e78f7d2a1aa\"}]},\"type\":\"ConnectorPlacement.EquallySpacedConnector\",\"uuid\":\"7dd7fe03-b221-4701-a7b2-6552f08320da\"}],\"packageUris\":[\"http://schema.mathworks.com/mf0/Connector/R2020b\"],\"version\":\"1.0\"}"
  multa4 : My_FI_Operations/multa4_  SystemSampleTime=-1  VariantActivationTime=update diagram  Latency=0  AutoFrameSizeCalculation=off
      settings: PortSchema="{\"entries\":[{\"content\":{\"sides\":[{\"content\":{\"connectorIds\":[\"In1\"]},\"type\":\"ConnectorPlacement.EquallySpacedRectSide\",\"uuid\":\"423828e0-6700-4575-ac06-a5fb7cb5569f\"},{\"content\":{\"connectorIds\":[],\"side\":\"RIGHT\"},\"type\":\"ConnectorPlacement.EquallySpacedRectSide\",\"uuid\":\"a42db842-eb55-44f2-8f04-0144bc45d908\"},{\"content\":{\"connectorIds\":[\"In2\"],\"side\":\"TOP\"},\"type\":\"ConnectorPlacement.EquallySpacedRectSide\",\"uuid\":\"eef5137d-31f0-46b4-a53b-5aa31464a7f9\"},{\"content\":{\"connectorIds\":[\"Out1\"],\"side\":\"BOTTOM\"},\"type\":\"ConnectorPlacement.EquallySpacedRectSide\",\"uuid\":\"24a9476e-4370-431a-bbc5-245c90c7a6e7\"}]},\"type\":\"ConnectorPlacement.EquallySpacedConnector\",\"uuid\":\"7dd7fe03-b221-4701-a7b2-6552f08320da\"}],\"packageUris\":[\"http://schema.mathworks.com/mf0/Connector/R2020b\"],\"version\":\"1.0\"}"
  multa6 : My_FI_Operations/multa6_  SystemSampleTime=-1  VariantActivationTime=update diagram  Latency=0  AutoFrameSizeCalculation=off
      settings: PortSchema="{\"entries\":[{\"content\":{\"sides\":[{\"content\":{\"connectorIds\":[\"In1\"]},\"type\":\"ConnectorPlacement.EquallySpacedRectSide\",\"uuid\":\"423828e0-6700-4575-ac06-a5fb7cb5569f\"},{\"content\":{\"connectorIds\":[],\"side\":\"RIGHT\"},\"type\":\"ConnectorPlacement.EquallySpacedRectSide\",\"uuid\":\"a42db842-eb55-44f2-8f04-0144bc45d908\"},{\"content\":{\"connectorIds\":[\"In2\"],\"side\":\"TOP\"},\"type\":\"ConnectorPlacement.EquallySpacedRectSide\",\"uuid\":\"eef5137d-31f0-46b4-a53b-5aa31464a7f9\"},{\"content\":{\"connectorIds\":[\"Out1\"],\"side\":\"BOTTOM\"},\"type\":\"ConnectorPlacement.EquallySpacedRectSide\",\"uuid\":\"47329aef-84bb-47a0-9b32-b12909a392a1\"}]},\"type\":\"ConnectorPlacement.EquallySpacedConnector\",\"uuid\":\"7dd7fe03-b221-4701-a7b2-6552f08320da\"}],\"packageUris\":[\"http://schema.mathworks.com/mf0/Connector/R2020b\"],\"version\":\"1.0\"}"
  multa8 : My_FI_Operations/multa8_  SystemSampleTime=-1  VariantActivationTime=update diagram  Latency=0  AutoFrameSizeCalculation=off
      settings: PortSchema="{\"entries\":[{\"content\":{\"sides\":[{\"content\":{\"connectorIds\":[\"In1\"]},\"type\":\"ConnectorPlacement.EquallySpacedRectSide\",\"uuid\":\"423828e0-6700-4575-ac06-a5fb7cb5569f\"},{\"content\":{\"connectorIds\":[],\"side\":\"RIGHT\"},\"type\":\"ConnectorPlacement.EquallySpacedRectSide\",\"uuid\":\"a42db842-eb55-44f2-8f04-0144bc45d908\"},{\"content\":{\"connectorIds\":[\"In2\"],\"side\":\"TOP\"},\"type\":\"ConnectorPlacement.EquallySpacedRectSide\",\"uuid\":\"eef5137d-31f0-46b4-a53b-5aa31464a7f9\"},{\"content\":{\"connectorIds\":[\"Out1\"],\"side\":\"BOTTOM\"},\"type\":\"ConnectorPlacement.EquallySpacedRectSide\",\"uuid\":\"5c073f60-f22f-4cd7-abc5-d0d5f88f0213\"}]},\"type\":\"ConnectorPlacement.EquallySpacedConnector\",\"uuid\":\"7dd7fe03-b221-4701-a7b2-6552f08320da\"}],\"packageUris\":[\"http://schema.mathworks.com/mf0/Connector/R2020b\"],\"version\":\"1.0\"}"
  suma2 : My_FI_Operations/suma2_  SystemSampleTime=-1  VariantActivationTime=update diagram  Latency=0  AutoFrameSizeCalculation=off
      settings: PortSchema="{\"entries\":[{\"content\":{\"sides\":[{\"content\":{\"connectorIds\":[\"Out1\"]},\"type\":\"ConnectorPlacement.EquallySpacedRectSide\",\"uuid\":\"423828e0-6700-4575-ac06-a5fb7cb5569f\"},{\"content\":{\"connectorIds\":[\"In2\"],\"side\":\"RIGHT\"},\"type\":\"ConnectorPlacement.EquallySpacedRectSide\",\"uuid\":\"a42db842-eb55-44f2-8f04-0144bc45d908\"},{\"content\":{\"connectorIds\":[\"In1\"],\"side\":\"TOP\"},\"type\":\"ConnectorPlacement.EquallySpacedRectSide\",\"uuid\":\"eef5137d-31f0-46b4-a53b-5aa31464a7f9\"}]},\"type\":\"ConnectorPlacement.EquallySpacedConnector\",\"uuid\":\"7dd7fe03-b221-4701-a7b2-6552f08320da\"}],\"packageUris\":[\"http://schema.mathworks.com/mf0/Connector/R2020b\"],\"version\":\"1.0\"}"
  suma4 : My_FI_Operations/suma4_  SystemSampleTime=-1  VariantActivationTime=update diagram  Latency=0  AutoFrameSizeCalculation=off
      settings: PortSchema="{\"entries\":[{\"content\":{\"sides\":[{\"content\":{\"connectorIds\":[\"Out1\"]},\"type\":\"ConnectorPlacement.EquallySpacedRectSide\",\"uuid\":\"423828e0-6700-4575-ac06-a5fb7cb5569f\"},{\"content\":{\"connectorIds\":[\"In2\"],\"side\":\"RIGHT\"},\"type\":\"ConnectorPlacement.EquallySpacedRectSide\",\"uuid\":\"a42db842-eb55-44f2-8f04-0144bc45d908\"},{\"content\":{\"connectorIds\":[\"In1\"],\"side\":\"TOP\"},\"type\":\"ConnectorPlacement.EquallySpacedRectSide\",\"uuid\":\"eef5137d-31f0-46b4-a53b-5aa31464a7f9\"}]},\"type\":\"ConnectorPlacement.EquallySpacedConnector\",\"uuid\":\"7dd7fe03-b221-4701-a7b2-6552f08320da\"}],\"packageUris\":[\"http://schema.mathworks.com/mf0/Connector/R2020b\"],\"version\":\"1.0\"}"
  suma6 : My_FI_Operations/suma6_  SystemSampleTime=-1  VariantActivationTime=update diagram  Latency=0  AutoFrameSizeCalculation=off
      settings: PortSchema="{\"entries\":[{\"content\":{\"sides\":[{\"content\":{\"connectorIds\":[\"Out1\"]},\"type\":\"ConnectorPlacement.EquallySpacedRectSide\",\"uuid\":\"423828e0-6700-4575-ac06-a5fb7cb5569f\"},{\"content\":{\"connectorIds\":[\"In2\"],\"side\":\"RIGHT\"},\"type\":\"ConnectorPlacement.EquallySpacedRectSide\",\"uuid\":\"a42db842-eb55-44f2-8f04-0144bc45d908\"},{\"content\":{\"connectorIds\":[\"In1\"],\"side\":\"TOP\"},\"type\":\"ConnectorPlacement.EquallySpacedRectSide\",\"uuid\":\"eef5137d-31f0-46b4-a53b-5aa31464a7f9\"}]},\"type\":\"ConnectorPlacement.EquallySpacedConnector\",\"uuid\":\"7dd7fe03-b221-4701-a7b2-6552f08320da\"}],\"packageUris\":[\"http://schema.mathworks.com/mf0/Connector/R2020b\"],\"version\":\"1.0\"}"
  sumd : My_FI_Operations/sumd-2_  SystemSampleTime=-1  VariantActivationTime=update diagram  Latency=0  AutoFrameSizeCalculation=off
      settings: PortSchema="{\"entries\":[{\"content\":{\"sides\":[{\"content\":{\"connectorIds\":[]},\"type\":\"ConnectorPlacement.EquallySpacedRectSide\",\"uuid\":\"423828e0-6700-4575-ac06-a5fb7cb5569f\"},{\"content\":{\"connectorIds\":[\"In2\"],\"side\":\"RIGHT\"},\"type\":\"ConnectorPlacement.EquallySpacedRectSide\",\"uuid\":\"a42db842-eb55-44f2-8f04-0144bc45d908\"},{\"content\":{\"connectorIds\":[\"Out1\"],\"side\":\"TOP\"},\"type\":\"ConnectorPlacement.EquallySpacedRectSide\",\"uuid\":\"eef5137d-31f0-46b4-a53b-5aa31464a7f9\"},{\"content\":{\"connectorIds\":[\"In1\"],\"side\":\"BOTTOM\"},\"type\":\"ConnectorPlacement.EquallySpacedRectSide\",\"uuid\":\"0a29e77a-4bdf-45d0-8a25-1103c3446174\"}]},\"type\":\"ConnectorPlacement.EquallySpacedConnector\",\"uuid\":\"7dd7fe03-b221-4701-a7b2-6552f08320da\"}],\"packageUris\":[\"http://schema.mathworks.com/mf0/Connector/R2020b\"],\"version\":\"1.0\"}"
  sumin : My_FI_Operations/sumin_  SystemSampleTime=-1  VariantActivationTime=update diagram  Latency=0  AutoFrameSizeCalculation=off
      settings: PortSchema="{\"entries\":[{\"content\":{\"sides\":[{\"content\":{\"connectorIds\":[\"In1\"]},\"type\":\"ConnectorPlacement.EquallySpacedRectSide\",\"uuid\":\"423828e0-6700-4575-ac06-a5fb7cb5569f\"},{\"content\":{\"connectorIds\":[\"Out1\"],\"side\":\"RIGHT\"},\"type\":\"ConnectorPlacement.EquallySpacedRectSide\",\"uuid\":\"a42db842-eb55-44f2-8f04-0144bc45d908\"},{\"content\":{\"connectorIds\":[],\"side\":\"TOP\"},\"type\":\"ConnectorPlacement.EquallySpacedRectSide\",\"uuid\":\"eef5137d-31f0-46b4-a53b-5aa31464a7f9\"},{\"content\":{\"connectorIds\":[\"In2\"],\"side\":\"BOTTOM\"},\"type\":\"ConnectorPlacement.EquallySpacedRectSide\",\"uuid\":\"f3760898-0e2b-4385-8757-2cc61988fa54\"}]},\"type\":\"ConnectorPlacement.EquallySpacedConnector\",\"uuid\":\"7dd7fe03-b221-4701-a7b2-6552f08320da\"}],\"packageUris\":[\"http://schema.mathworks.com/mf0/Connector/R2020b\"],\"version\":\"1.0\"}"
  sumq : My_FI_Operations/sumq-1_  SystemSampleTime=-1  VariantActivationTime=update diagram  Latency=0  AutoFrameSizeCalculation=off
      settings: PortSchema="{\"entries\":[{\"content\":{\"sides\":[{\"content\":{\"connectorIds\":[]},\"type\":\"ConnectorPlacement.EquallySpacedRectSide\",\"uuid\":\"423828e0-6700-4575-ac06-a5fb7cb5569f\"},{\"content\":{\"connectorIds\":[\"In2\"],\"side\":\"RIGHT\"},\"type\":\"ConnectorPlacement.EquallySpacedRectSide\",\"uuid\":\"a42db842-eb55-44f2-8f04-0144bc45d908\"},{\"content\":{\"connectorIds\":[\"Out1\"],\"side\":\"TOP\"},\"type\":\"ConnectorPlacement.EquallySpacedRectSide\",\"uuid\":\"eef5137d-31f0-46b4-a53b-5aa31464a7f9\"},{\"content\":{\"connectorIds\":[\"In1\"],\"side\":\"BOTTOM\"},\"type\":\"ConnectorPlacement.EquallySpacedRectSide\",\"uuid\":\"2873f229-5340-47da-9b40-109923f96826\"}]},\"type\":\"ConnectorPlacement.EquallySpacedConnector\",\"uuid\":\"7dd7fe03-b221-4701-a7b2-6552f08320da\"}],\"packageUris\":[\"http://schema.mathworks.com/mf0/Connector/R2020b\"],\"version\":\"1.0\"}"
  Out1 : Outport
  Out2 : Outport  Port=2
  Out3 : Outport  Port=3
  wires:
  suma4/1 -> Out2/1
  suma2/1 -> Out3/1
  In3/1 -> sumd/1
  In1/1 -> Delay0/1
  In2/1 -> sumq/2
  a6/1 -> multa6/1
  sumq/1 -> sumin/2
  multa8/1 -> Delay22/1
  multa10/1 -> Delay12/1
  Delay11/1 -> suma4/2
  suma6/1 -> Delay32/1
  a8/1 -> multa8/1
  Delay34/1 -> Delay33/1
  multa2/1 -> suma2/1
  multa12/1 -> Delay34/1
  a4/1 -> multa4/1
  a10/1 -> multa10/1
  multa6/1 -> suma6/1
  ZOH/1 -> Out1/1
  Delay12/1 -> Delay11/1
  multa4/1 -> suma4/1
  a2/1 -> multa2/1
  sumd/1 -> sumq/1
  Delay21/1 -> suma2/2
  Delay32/1 -> Delay31/1
  Delay33/1 -> suma6/2
  sumin/1 -> ZOH/1, multa12/2, multa10/2, multa8/2, multa6/2, multa4/2, multa2/2
  Delay31/1 -> sumd/2
  Delay22/1 -> Delay21/1
  a12/1 -> multa12/1
  Delay0/1 -> sumin/1

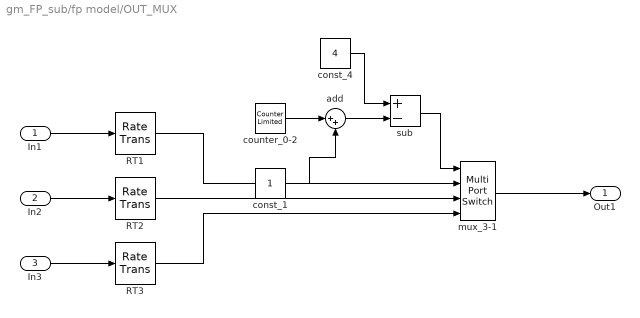
== system gm_FP_sub/fp model/OUT_MUX ==
  In1 : Inport
  In2 : Inport  Port=2
  In3 : Inport  Port=3
  RT1 : RateTransition  OutPortSampleTime=Ts
  RT2 : RateTransition  OutPortSampleTime=Ts
  RT3 : RateTransition  OutPortSampleTime=Ts
  add : Sum  Inputs=|++  OutDataTypeStr=fixdt(0,2,0)
  const_1 : Constant  OutDataTypeStr=fixdt(0,1,0)
  const_4 : Constant  Value=4  OutDataTypeStr=fixdt(0,3,0)
  counter_0-2 : simulink/Sources/Counter Limited  uplimit=2  tsamp=Ts
  mux_3-1 : MultiPortSwitch  OutDataTypeStr=fixdt(1,WL,FLout)  RndMeth=Nearest  SaturateOnIntegerOverflow=off  InputSameDT=off
  sub : Sum  Inputs=+-  OutDataTypeStr=fixdt(0,2,0)
  Out1 : Outport
  wires:
  In3/1 -> RT3/1
  mux_3-1/1 -> Out1/1
  In1/1 -> RT1/1
  In2/1 -> RT2/1
  RT2/1 -> mux_3-1/3
  RT1/1 -> mux_3-1/2
  const_4/1 -> sub/1
  add/1 -> sub/2
  counter_0-2/1 -> add/1
  sub/1 -> mux_3-1/1
  const_1/1 -> add/2
  RT3/1 -> mux_3-1/4

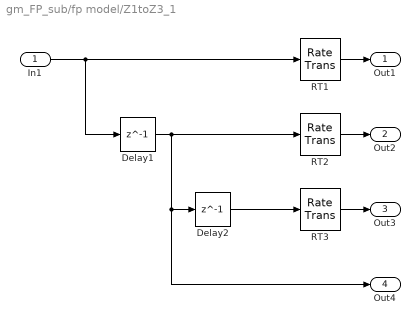
== system gm_FP_sub/fp model/Z1toZ3_1 ==
  In1 : Inport
  Delay1 : Delay  DelayLength=1  SampleTime=Ts
  Delay2 : Delay  DelayLength=1  SampleTime=Ts
  RT1 : RateTransition  OutPortSampleTime=3*Ts
  RT2 : RateTransition  OutPortSampleTime=3*Ts
  RT3 : RateTransition  OutPortSampleTime=3*Ts
  Out1 : Outport
  Out2 : Outport  Port=2
  Out3 : Outport  Port=3
  Out4 : Outport  Port=4
  wires:
  RT3/1 -> Out3/1
  RT2/1 -> Out2/1
  RT1/1 -> Out1/1
  In1/1 -> RT1/1, Delay1/1
  Delay2/1 -> RT3/1
  Delay1/1 -> Delay2/1, Out4/1, RT2/1

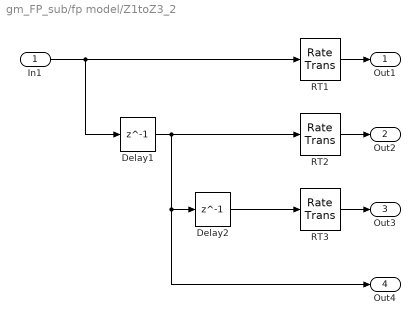
== system gm_FP_sub/fp model/Z1toZ3_2 ==
  In1 : Inport
  Delay1 : Delay  DelayLength=1  SampleTime=Ts
  Delay2 : Delay  DelayLength=1  SampleTime=Ts
  RT1 : RateTransition  OutPortSampleTime=3*Ts
  RT2 : RateTransition  OutPortSampleTime=3*Ts
  RT3 : RateTransition  OutPortSampleTime=3*Ts
  Out1 : Outport
  Out2 : Outport  Port=2
  Out3 : Outport  Port=3
  Out4 : Outport  Port=4
  wires:
  RT3/1 -> Out3/1
  RT2/1 -> Out2/1
  RT1/1 -> Out1/1
  In1/1 -> RT1/1, Delay1/1
  Delay2/1 -> RT3/1
  Delay1/1 -> Delay2/1, Out4/1, RT2/1

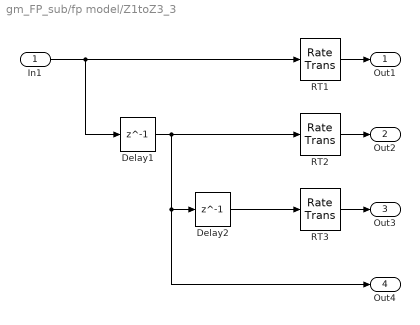
== system gm_FP_sub/fp model/Z1toZ3_3 ==
  In1 : Inport
  Delay1 : Delay  DelayLength=1  SampleTime=Ts
  Delay2 : Delay  DelayLength=1  SampleTime=Ts
  RT1 : RateTransition  OutPortSampleTime=3*Ts
  RT2 : RateTransition  OutPortSampleTime=3*Ts
  RT3 : RateTransition  OutPortSampleTime=3*Ts
  Out1 : Outport
  Out2 : Outport  Port=2
  Out3 : Outport  Port=3
  Out4 : Outport  Port=4
  wires:
  RT3/1 -> Out3/1
  RT2/1 -> Out2/1
  RT1/1 -> Out1/1
  In1/1 -> RT1/1, Delay1/1
  Delay2/1 -> RT3/1
  Delay1/1 -> Delay2/1, Out4/1, RT2/1
